simulink model "ACtoDC_WPT_current_control"  (R2018a)
settings: Solver=FixedStepAuto  StartTime=0.0  StopTime=stopTime  FixedStep=sampleTime  RelTol=1e-3
InitFcn:
  | fs=150e3; %Hz
  | wo=2*pi*fs;
  | stopTime=0.1;
  | sampleTime=1e-8;
  | deadtime= round(((1/fs)/20)/sampleTime);
  | Vdc=100;
  | Lp=82e-6;
  | Ls=66e-6;
  | Cs=1/ (Ls*4*pi*pi*150e3*150e3);
  | Cp=1/ (Lp*4*pi*pi*150e3*150e3);
  | Cp=Cp*5;
  | Rp=0.3;
  | Rs=0.2;
  | RLOAD=20
  | k=0.2;
  | M=sqrt(Lp*Ls)*k;
  | Cout=1e-6; %F
  | C2=(Lp-(1/(wo^2*Cp)))/((wo^4*M^4/RLOAD)+(wo^2*(Lp-(1/(wo^2*Cs)))^2))
libraries: powerlib x29, simulink x1
settings Model: Creator=enes_  LastModifiedBy=enes_

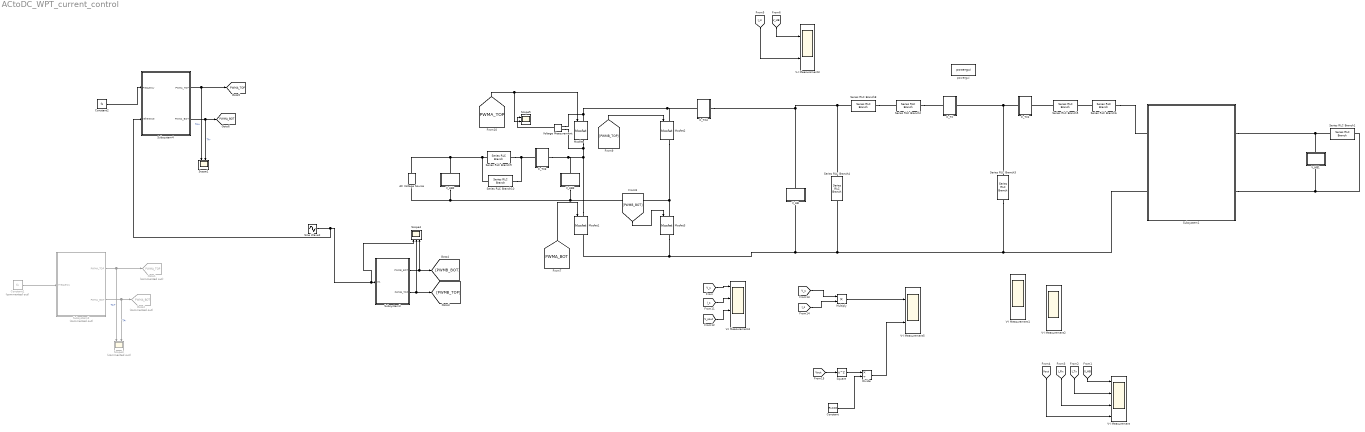
== system ACtoDC_WPT_current_control ==
  AC Voltage Source : powerlib/Electrical Sources/AC Voltage Source  Amplitude=100  Phase=0  Frequency=50  SampleTime=0  Measurements=None  BusType=swing  Pref=10e3  Qref=0  Qmin=-inf  Qmax=+inf
  C_TX : Subsystem
  C_TX1 : Subsystem
  C_TX3 : Subsystem
  C_TX4 : Subsystem
  Constant : Constant  Value=RLOAD
  Constant1 : Constant  Commented=on  Value=fs
  Constant2 : Constant  Value=fs
  Divide : Product  Inputs=*/
  Goto1 : Goto  Commented=on  GotoTag=PWMA_TOP  TagVisibility=global
  Goto2 : Goto  Commented=on  GotoTag=PWMA_BOT  TagVisibility=global
  Mosfet{,1..3} (4 alike) : powerlib/Power Electronics/Mosfet  Ron=0.1  Lon=0  Rd=0.01  Vfd=0  IC=0  Rs=1e5  Cs=inf  Measurements=on
  Multiply : Product
  Scope1 : Scope  NumInputPorts=2
  Scope3 : Scope  Commented=on  NumInputPorts=2
  Scope4 : Scope  NumInputPorts=3
  Scope5 : Scope  NumInputPorts=2
  Series RLC Branch1 : powerlib/Elements/Series RLC Branch  LConnTagsString=__new0  RConnTagsString=__new0  BranchType=R  Resistance=RLOAD  Inductance=Lp  SetiL0=off  InitialCurrent=0  Capacitance=Cp  Setx0=off  InitialVoltage=0  Measurements=None
  Series RLC Branch10 : powerlib/Elements/Series RLC Branch  LConnTagsString=__new0  RConnTagsString=__new0  BranchType=R  Resistance=10e3  Inductance=10e3  SetiL0=off  InitialCurrent=0  Capacitance=Cp  Setx0=off  InitialVoltage=0  Measurements=None
  Series RLC Branch2 : powerlib/Elements/Series RLC Branch  LConnTagsString=__new0  RConnTagsString=__new0  BranchType=L  Resistance=Rp  Inductance=Lp-M  SetiL0=off  InitialCurrent=0  Capacitance=Cp  Setx0=off  InitialVoltage=0  Measurements=None
  Series RLC Branch3 : powerlib/Elements/Series RLC Branch  LConnTagsString=__new0  RConnTagsString=__new0  BranchType=L  Resistance=Rp  Inductance=M  SetiL0=off  InitialCurrent=0  Capacitance=Cp  Setx0=off  InitialVoltage=0  Measurements=None
  Series RLC Branch4 : powerlib/Elements/Series RLC Branch  LConnTagsString=__new0  RConnTagsString=__new0  BranchType=C  Resistance=Rp  Inductance=Lp  SetiL0=off  InitialCurrent=0  Capacitance=C2  Setx0=off  InitialVoltage=0  Measurements=None
  Series RLC Branch5 : powerlib/Elements/Series RLC Branch  LConnTagsString=__new0  RConnTagsString=__new0  BranchType=L  Resistance=Rp  Inductance=Ls-M  SetiL0=off  InitialCurrent=0  Capacitance=Cp  Setx0=off  InitialVoltage=0  Measurements=None
  Series RLC Branch6 : powerlib/Elements/Series RLC Branch  LConnTagsString=__new0  RConnTagsString=__new0  BranchType=C  Resistance=Rp  Inductance=Lp  SetiL0=off  InitialCurrent=0  Capacitance=Cs  Setx0=off  InitialVoltage=0  Measurements=None
  Series RLC Branch8 : powerlib/Elements/Series RLC Branch  LConnTagsString=__new0  RConnTagsString=__new0  BranchType=C  Resistance=Rp  Inductance=Lp  SetiL0=off  InitialCurrent=0  Capacitance=Cp  Setx0=off  InitialVoltage=0  Measurements=None
  Series RLC Branch9 : powerlib/Elements/Series RLC Branch  LConnTagsString=__new0  RConnTagsString=__new0  BranchType=L  Resistance=Rp  Inductance=100e-6  SetiL0=off  InitialCurrent=0  Capacitance=Cp  Setx0=off  InitialVoltage=0  Measurements=None
  Sine Wave2 : Sin  Amplitude=pi/2  Frequency=2*pi*50  SampleTime=0
  Square : Math  Operator=square  SaturateOnIntegerOverflow=on
  Subsystem1 : Subsystem
  Subsystem2 : Subsystem  Commented=on
  Subsystem3 : Subsystem
  Subsystem4 : Subsystem
  V-I Measurement : Scope  NumInputPorts=4
  V-I Measurement1 : Scope  NumInputPorts=4
  V-I Measurement2 : Scope  NumInputPorts=2
  V-I Measurement3 : Scope  NumInputPorts=2
  V-I Measurement4 : Scope  NumInputPorts=4
  V-I Measurement5 : Scope  NumInputPorts=2
  V_HB : Subsystem
  V_HB1 : Subsystem
  V_HB2 : Subsystem
  V_HB3 : Subsystem
  Voltage Measurement : powerlib/Measurements/Voltage Measurement  PhasorSimulation=off  OutputType=Complex  PSBequivalent=0
  powergui : powerlib/powergui  Priority=1  SimulationMode=Discrete  SampleTime=sampleTime  frequency=60  Iterations=50  frequencyindice=0  Pbase=100e6  ErrMax=1e-4  UnitsV=kV  UnitsW=MW  buscounter=0  FunctionMessages=off  echomessages=off  EnableUseOfTLC=off  CurrentSourceSwitches=off  DisableSnubberDevices=off  DisableRonSwitches=off  DisableVfSwitches=off  DisplayEquations=off  SolverType=Tustin/Backward Euler (TBE)  Interpol=off  ExternalGateDelay=off  methode=off  Ts=100  x0status=blocks  SPID=off  SwTol=0  HookPort=off  RestoreLinks=warning  ResistiveCurrentMeasurement=off  Frange=[0:2:500]  Ylog=off  Xlog=on  ShowGrid=off  save=off  variable=ZData  structure=ScopeData2  ZoomFFT=off  StartTime=0.0  cycles=4  DisplayStyle=2  fundamental=100  FreqAxis=off  MaxFrequency=600e3  frequencyindicesteady=1  RmsSteady=1  display=off
  tag scope: PWMA_BOT=global, PWMA_TOP=global
  wires:
  [V_HB] -> V-I Measurement/1
  [I_Tx] -> V-I Measurement/2
  [I_Rx] -> V-I Measurement/3
  [Vout] -> V-I Measurement/4
  [V_HB] -> V-I Measurement3/1
  [I_in] -> V-I Measurement3/2
  [PWMA_TOP] -> Scope5/2, Mosfet/1
  Subsystem3/1(PWMB_BOT) -> [PWMB_BOT], Scope4/3
  Subsystem3/2(PWMB_TOP) -> [PWMB_TOP], Scope4/2
  [PWMB_TOP] -> Mosfet2/1
  [PWMA_BOT] -> Mosfet1/1
  [PWMB_BOT] -> Mosfet3/1
  Voltage Measurement/1 -> Scope5/1
  Subsystem2/2(PWMA_BOT) -> Goto2/1, Scope3/2  "TA-"
  Constant1/1 -> Subsystem2/1(Frequency)
  Sine Wave2/1 -> Subsystem4/2(refrerence), Scope4/1, Subsystem3/1(In1)
  Subsystem2/1(PWMA_TOP) -> Goto1/1, Scope3/1  "TA+"
  [V_s] -> V-I Measurement4/1
  [I_s] -> V-I Measurement4/2
  [V_sout] -> V-I Measurement4/3
  [V_s] -> Multiply/1
  [I_s] -> Multiply/2
  Multiply/1 -> V-I Measurement5/1
  [Vout] -> Square/1
  Square/1 -> Divide/1
  Constant/1 -> Divide/2
  Divide/1 -> V-I Measurement5/2
  Subsystem4/1(PWMA_TOP) -> [PWMA_TOP], Scope1/1  "TA+"
  Subsystem4/2(PWMA_BOT) -> [PWMA_BOT], Scope1/2  "TA-"
  Constant2/1 -> Subsystem4/1(Frequency)
  connections:
  Subsystem1/RConn2 -- V_HB1/LConn1 -- Series RLC Branch1/LConn1
  Mosfet3/RConn1 -- Series RLC Branch3/RConn1 -- Subsystem1/LConn2 -- Series RLC Branch4/RConn1 -- V_HB/LConn1 -- Mosfet1/RConn1
  Series RLC Branch5/LConn1 -- C_TX1/RConn1
  Series RLC Branch2/RConn1 -- C_TX/LConn1
  Series RLC Branch6/LConn1 -- Series RLC Branch5/RConn1
  Series RLC Branch6/RConn1 -- Subsystem1/LConn1
  Series RLC Branch3/LConn1 -- C_TX1/LConn1 -- C_TX/RConn1
  Series RLC Branch1/RConn1 -- Subsystem1/RConn1 -- V_HB1/RConn1
  Mosfet1/LConn1 -- V_HB3/RConn1 -- C_TX3/RConn1 -- Mosfet/RConn1 -- Voltage Measurement/LConn2
  V_HB2/LConn1 -- AC Voltage Source/LConn1 -- Mosfet2/RConn1 -- Mosfet3/LConn1 -- V_HB3/LConn1
  Series RLC Branch9/RConn1 -- Series RLC Branch10/RConn1 -- C_TX3/LConn1
  V_HB/RConn1 -- C_TX4/RConn1 -- Series RLC Branch8/RConn1 -- Series RLC Branch4/LConn1
  Voltage Measurement/LConn1 -- C_TX4/LConn1 -- Mosfet2/LConn1 -- Mosfet/LConn1
  Series RLC Branch8/LConn1 -- Series RLC Branch2/LConn1
  V_HB2/RConn1 -- AC Voltage Source/RConn1 -- Series RLC Branch10/LConn1 -- Series RLC Branch9/LConn1

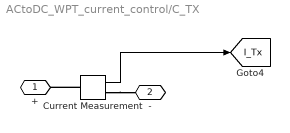
== system ACtoDC_WPT_current_control/C_TX ==
  Current Measurement : powerlib/Measurements/Current Measurement  PhasorSimulation=off  OutputType=Complex  PSBequivalent=0
  + : PMIOPort  Side=Left
  - : PMIOPort  Port=2  Side=Right
  tag scope: I_Tx=global
  wires:
  Current Measurement/1 -> [I_Tx]
  connections:
  Current Measurement/RConn1 -- -/RConn1
  Current Measurement/LConn1 -- +/RConn1

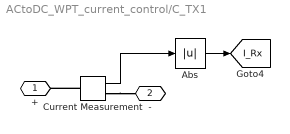
== system ACtoDC_WPT_current_control/C_TX1 ==
  Abs : Abs
  Current Measurement : powerlib/Measurements/Current Measurement  PhasorSimulation=off  OutputType=Complex  PSBequivalent=0
  + : PMIOPort  Side=Left
  - : PMIOPort  Port=2  Side=Right
  tag scope: I_Rx=global
  wires:
  Current Measurement/1 -> Abs/1
  Abs/1 -> [I_Rx]
  connections:
  Current Measurement/RConn1 -- -/RConn1
  Current Measurement/LConn1 -- +/RConn1

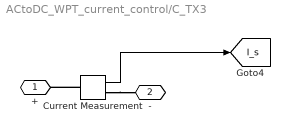
== system ACtoDC_WPT_current_control/C_TX3 ==
  Current Measurement : powerlib/Measurements/Current Measurement  PhasorSimulation=off  OutputType=Complex  PSBequivalent=0
  + : PMIOPort  Side=Left
  - : PMIOPort  Port=2  Side=Right
  tag scope: I_s=global
  wires:
  Current Measurement/1 -> [I_s]
  connections:
  Current Measurement/RConn1 -- -/RConn1
  Current Measurement/LConn1 -- +/RConn1

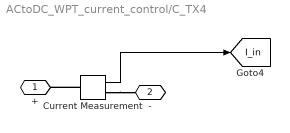
== system ACtoDC_WPT_current_control/C_TX4 ==
  Current Measurement : powerlib/Measurements/Current Measurement  PhasorSimulation=off  OutputType=Complex  PSBequivalent=0
  + : PMIOPort  Side=Left
  - : PMIOPort  Port=2  Side=Right
  tag scope: I_in=global
  wires:
  Current Measurement/1 -> [I_in]
  connections:
  Current Measurement/RConn1 -- -/RConn1
  Current Measurement/LConn1 -- +/RConn1

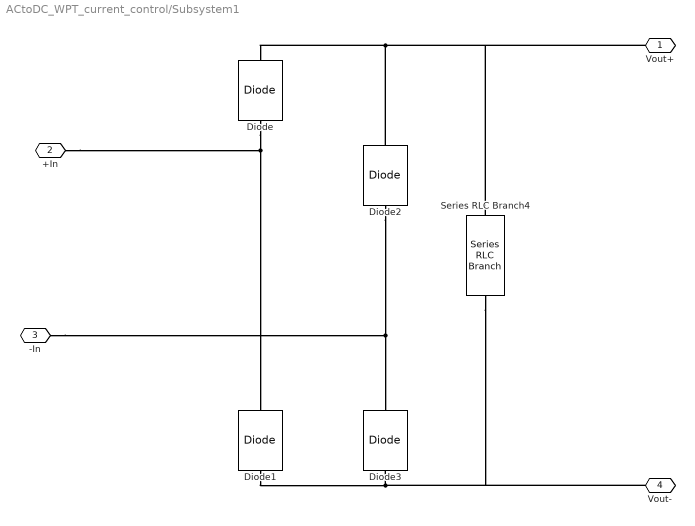
== system ACtoDC_WPT_current_control/Subsystem1 ==
  Diode{,1..3} (4 alike) : powerlib/Power Electronics/Diode  Ron=0.001  Lon=0  Vf=0.8  IC=0  UseSnubber=0  Rs=500  Cs=250e-9  Measurements=off
  Series RLC Branch4 : powerlib/Elements/Series RLC Branch  LConnTagsString=__new0  RConnTagsString=__new0  BranchType=C  Resistance=RLOAD  Inductance=Lp  SetiL0=off  InitialCurrent=0  Capacitance=Cout  Setx0=off  InitialVoltage=0  Measurements=None
  Vout+ : PMIOPort  Side=Right
  +In : PMIOPort  Port=2  Side=Left
  -In : PMIOPort  Port=3  Side=Left
  Vout- : PMIOPort  Port=4  Side=Right
  connections:
  Diode/LConn1 -- +In/RConn1 -- Diode1/RConn1
  Vout+/RConn1 -- Series RLC Branch4/LConn1 -- Diode/RConn1 -- Diode2/RConn1
  -In/RConn1 -- Diode3/RConn1 -- Diode2/LConn1
  Vout-/RConn1 -- Series RLC Branch4/RConn1 -- Diode1/LConn1 -- Diode3/LConn1

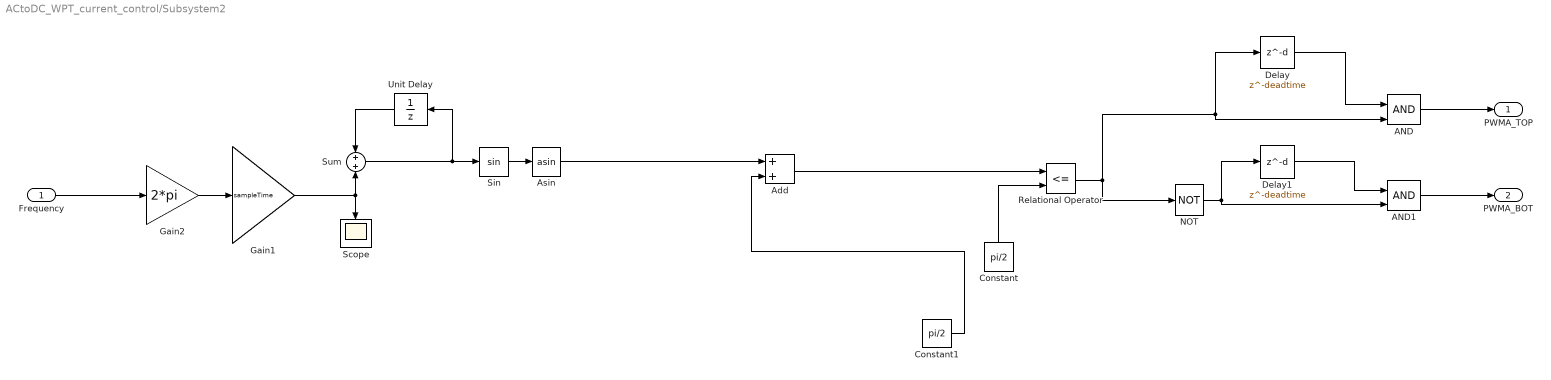
== system ACtoDC_WPT_current_control/Subsystem2 ==
  Frequency : Inport
  AND : Logic  IconShape=distinctive  AllPortsSameDT=off  OutDataTypeStr=boolean
  AND1 : Logic  IconShape=distinctive  AllPortsSameDT=off  OutDataTypeStr=boolean
  Add : Sum
  Asin : Trigonometry  Operator=asin
  Constant : Constant  Value=pi/2
  Constant1 : Constant  Value=pi/2
  Delay : Delay  DelayLength=deadtime
  Delay1 : Delay  DelayLength=deadtime
  Gain1 : Gain  Gain=sampleTime
  Gain2 : Gain  Gain=2*pi
  NOT : Logic  Operator=NOT  IconShape=distinctive  AllPortsSameDT=off  OutDataTypeStr=boolean
  Relational Operator : RelationalOperator  Operator=<=  OutDataTypeStr=boolean  RndMeth=Simplest
  Scope : Scope
  Sin : Trigonometry
  Sum : Sum
  Unit Delay : UnitDelay  SampleTime=-1
  PWMA_TOP : Outport
  PWMA_BOT : Outport  Port=2
  wires:
  Gain1/1 -> Sum/2, Scope/1
  AND/1 -> PWMA_TOP/1
  Asin/1 -> Add/1
  Sum/1 -> Sin/1, Unit Delay/1
  Gain2/1 -> Gain1/1
  Unit Delay/1 -> Sum/1
  Relational Operator/1 -> NOT/1, Delay/1, AND/2
  Frequency/1 -> Gain2/1
  Add/1 -> Relational Operator/1
  NOT/1 -> AND1/2, Delay1/1
  AND1/1 -> PWMA_BOT/1
  Delay/1 -> AND/1
  Delay1/1 -> AND1/1
  Sin/1 -> Asin/1
  Constant1/1 -> Add/2
  Constant/1 -> Relational Operator/2

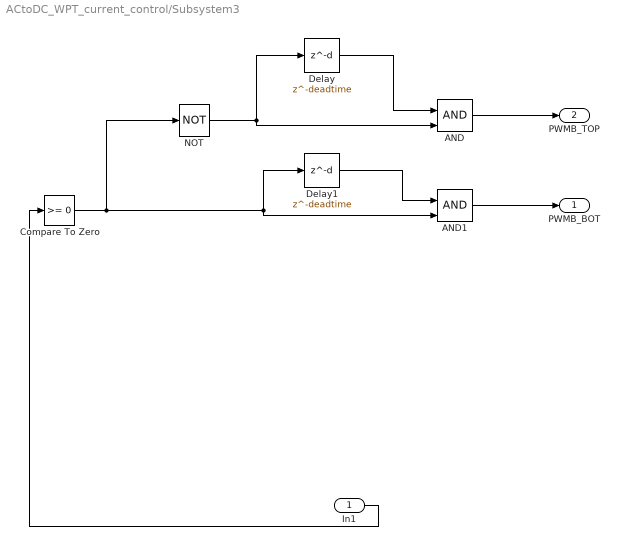
== system ACtoDC_WPT_current_control/Subsystem3 ==
  In1 : Inport
  AND : Logic  IconShape=distinctive  AllPortsSameDT=off  OutDataTypeStr=boolean
  AND1 : Logic  IconShape=distinctive  AllPortsSameDT=off  OutDataTypeStr=boolean
  Compare To Zero : simulink/Logic and Bit Operations/Compare To Zero  relop=>=  OutDataTypeStr=uint8
  Delay : Delay  DelayLength=deadtime
  Delay1 : Delay  DelayLength=deadtime
  NOT : Logic  Operator=NOT  IconShape=distinctive  AllPortsSameDT=off  OutDataTypeStr=boolean
  PWMB_BOT : Outport
  PWMB_TOP : Outport  Port=2
  wires:
  Delay1/1 -> AND1/1
  Delay/1 -> AND/1
  AND1/1 -> PWMB_BOT/1
  Compare To Zero/1 -> AND1/2, Delay1/1, NOT/1
  AND/1 -> PWMB_TOP/1
  In1/1 -> Compare To Zero/1
  NOT/1 -> Delay/1, AND/2

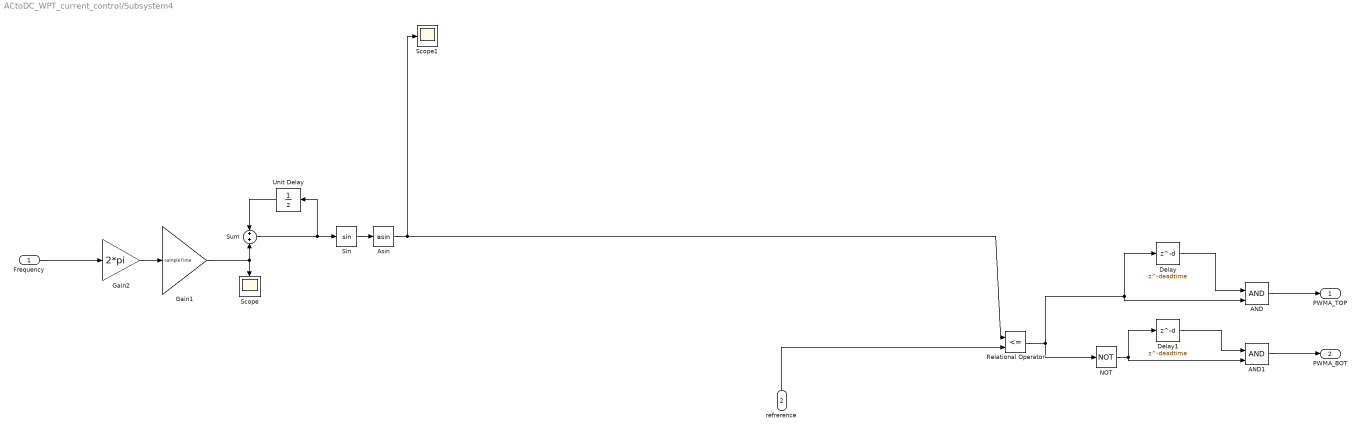
== system ACtoDC_WPT_current_control/Subsystem4 ==
  Frequency : Inport
  refrerence : Inport  Port=2
  AND : Logic  IconShape=distinctive  AllPortsSameDT=off  OutDataTypeStr=boolean
  AND1 : Logic  IconShape=distinctive  AllPortsSameDT=off  OutDataTypeStr=boolean
  Asin : Trigonometry  Operator=asin
  Delay : Delay  DelayLength=deadtime
  Delay1 : Delay  DelayLength=deadtime
  Gain1 : Gain  Gain=sampleTime
  Gain2 : Gain  Gain=2*pi
  NOT : Logic  Operator=NOT  IconShape=distinctive  AllPortsSameDT=off  OutDataTypeStr=boolean
  Relational Operator : RelationalOperator  Operator=<=  OutDataTypeStr=boolean  RndMeth=Simplest
  Scope : Scope
  Scope1 : Scope
  Sin : Trigonometry
  Sum : Sum
  Unit Delay : UnitDelay  SampleTime=-1
  PWMA_TOP : Outport
  PWMA_BOT : Outport  Port=2
  wires:
  Gain1/1 -> Sum/2, Scope/1
  Sum/1 -> Sin/1, Unit Delay/1
  Gain2/1 -> Gain1/1
  Unit Delay/1 -> Sum/1
  Frequency/1 -> Gain2/1
  Sin/1 -> Asin/1
  refrerence/1 -> Relational Operator/2
  Delay1/1 -> AND1/1
  AND/1 -> PWMA_TOP/1
  Delay/1 -> AND/1
  NOT/1 -> AND1/2, Delay1/1
  Asin/1 -> Relational Operator/1, Scope1/1
  AND1/1 -> PWMA_BOT/1
  Relational Operator/1 -> NOT/1, Delay/1, AND/2

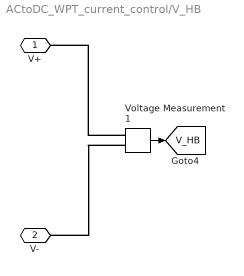
== system ACtoDC_WPT_current_control/V_HB ==
  Voltage Measurement1 : powerlib/Measurements/Voltage Measurement  PhasorSimulation=off  OutputType=Complex  PSBequivalent=0
  V+ : PMIOPort  Side=Right
  V- : PMIOPort  Port=2  Side=Left
  tag scope: V_HB=global
  wires:
  Voltage Measurement1/1 -> [V_HB]
  connections:
  Voltage Measurement1/LConn1 -- V+/RConn1
  Voltage Measurement1/LConn2 -- V-/RConn1

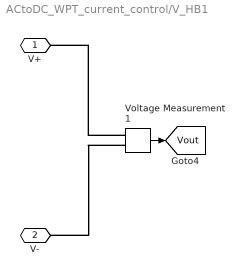
== system ACtoDC_WPT_current_control/V_HB1 ==
  Voltage Measurement1 : powerlib/Measurements/Voltage Measurement  PhasorSimulation=off  OutputType=Complex  PSBequivalent=0
  V+ : PMIOPort  Side=Right
  V- : PMIOPort  Port=2  Side=Left
  tag scope: Vout=global
  wires:
  Voltage Measurement1/1 -> [Vout]
  connections:
  Voltage Measurement1/LConn1 -- V+/RConn1
  Voltage Measurement1/LConn2 -- V-/RConn1

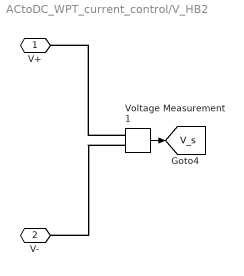
== system ACtoDC_WPT_current_control/V_HB2 ==
  Voltage Measurement1 : powerlib/Measurements/Voltage Measurement  PhasorSimulation=off  OutputType=Complex  PSBequivalent=0
  V+ : PMIOPort  Side=Right
  V- : PMIOPort  Port=2  Side=Left
  tag scope: V_s=global
  wires:
  Voltage Measurement1/1 -> [V_s]
  connections:
  Voltage Measurement1/LConn1 -- V+/RConn1
  Voltage Measurement1/LConn2 -- V-/RConn1

== system ACtoDC_WPT_current_control/V_HB3 ==
  Voltage Measurement1 : powerlib/Measurements/Voltage Measurement  PhasorSimulation=off  OutputType=Complex  PSBequivalent=0
  V+ : PMIOPort  Side=Right
  V- : PMIOPort  Port=2  Side=Left
  tag scope: V_sout=global
  wires:
  Voltage Measurement1/1 -> [V_sout]
  connections:
  Voltage Measurement1/LConn1 -- V+/RConn1
  Voltage Measurement1/LConn2 -- V-/RConn1
